simulink model "junta1_PD"  (R2020a)
settings: Solver=VariableStepAuto  StartTime=0.0  StopTime=9  RelTol=1e-3
values from neighbouring files (symbols this model uses):
  Kd = (2*xi*wn*Jeff - Beff)/Kl_eff    (= 0.005)    [identificacao_junta_1.m]
  Kl_eff = Kl*Beff    (= 2000)    [identificacao_junta_1.m]
  Kp = wn^2*Jeff/K    [identificacao_junta_1.m]
  N = 4    [identificacao_junta_1.m]
  T = 0.01    [identificacao_junta_1.m]
  Td = Kd/Kp    [identificacao_junta_1.m]
settings Model: Creator=fabio  LastModifiedBy=fabio

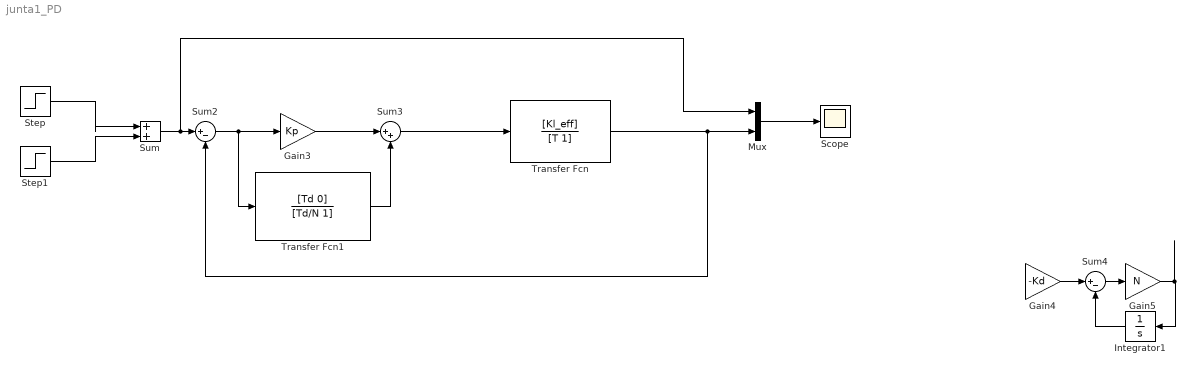
== system junta1_PD ==
  Gain3 : Gain  Gain=Kp
  Gain4 : Gain  Gain=-Kd
  Gain5 : Gain  Gain=N
  Integrator1 : Integrator
  Mux : Mux  Inputs=2
  Scope : Scope
  Step : Step  Time=3  After=5  SampleTime=0
  Step1 : Step  Time=6  After=4  SampleTime=0
  Sum : Sum  Inputs=|++
  Sum2 : Sum  Inputs=|+-
  Sum3 : Sum  Inputs=|++
  Sum4 : Sum  Inputs=|+-
  Transfer Fcn : TransferFcn  Numerator=[Kl_eff]  Denominator=[T 1]
  Transfer Fcn1 : TransferFcn  Numerator=[Td 0]  Denominator=[Td/N 1]
  wires:
  Sum2/1 -> Transfer Fcn1/1, Gain3/1
  Sum3/1 -> Transfer Fcn/1
  Transfer Fcn/1 -> Mux/2, Sum2/2
  Sum/1 -> Mux/1, Sum2/1
  Gain3/1 -> Sum3/1
  Step/1 -> Sum/1
  Step1/1 -> Sum/2
  Mux/1 -> Scope/1
  Sum4/1 -> Gain5/1
  ? -> Gain4/1
  Gain5/1 -> Integrator1/1
  Integrator1/1 -> Sum4/2
  Gain4/1 -> Sum4/1
  Transfer Fcn1/1 -> Sum3/2
